simulink library "Reynolds"  (Simulink 8.2)
settings: Solver=ode45  StartTime=0.0  StopTime=10.0  RelTol=1e-3
libraries: carnot x1
settings Model: Creator=lena.frank  LastModifiedBy=drhf

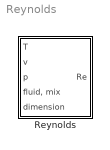
== system Reynolds ==
  Reynolds : Subsystem  mask(Reynolds number){}
      mask help:
      | Calculates the Reynolds number for a flow, give the characteristic dimension as an input.
      | Pipe: diameter
      | Duct: 4 * cross_section / perimeter
      | Plate: length
      mask Help: web(fullfile(path_carnot('help'),'Reynolds.html'),'-helpbrowser')

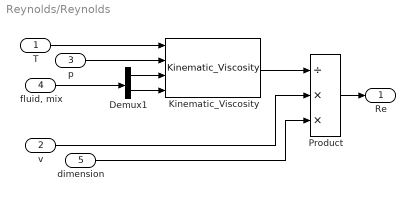
== system Reynolds/Reynolds ==
  T : Inport
  v : Inport  Port=2
  p : Inport  Port=3
  "fluid, mix" : Inport  Port=4
  dimension : Inport  Port=5
  Demux1 : Demux  Outputs=2
  Kinematic_Viscosity : carnot/Basic/Material_Properties/Kinematic_Viscosity  VariantControl=CarlibClassic  INPUTARGUMENTS=state variables (classic)  DEBUGLEVEL=WARNINGLEVEL  MAXTOTALMESSAGES=inf  MAXCONSECUTIVEMESSAGES=inf  WRITETOFILE=0  FILENAME='errors.txt'
  Product : Product  Inputs=/**  SaturateOnIntegerOverflow=on  InputSameDT=on  OutDataTypeStr=Inherit: Same as first input
  Re : Outport
  wires:
  Demux1/2 -> Kinematic_Viscosity/4
  Kinematic_Viscosity/1 -> Product/1
  "fluid, mix"/1 -> Demux1/1
  Demux1/1 -> Kinematic_Viscosity/3
  T/1 -> Kinematic_Viscosity/1
  p/1 -> Kinematic_Viscosity/2
  dimension/1 -> Product/3
  v/1 -> Product/2
  Product/1 -> Re/1
